simulink model "FOC_2"  (R2024a)
settings: Solver=FixedStepAuto  StartTime=0.0  StopTime=Inf  RelTol=1e-3  EnableMultiTasking=on
undefined symbols (not defined in the file): DiscIntNeverNeededParam, Down, GPTRIP1SEL, Ki, Ki_s, Kp, Kp_s, L, lambda, ma, p, T_period, TZ1, Up, Vdc
libraries: eeGeneralControl x6, simulink x6, c2837xDlib x5, c2802xlib x3
settings Model: ExtModeTrigDuration=8  Creator=kareem  LastModifiedBy=kareem
settings SolverCC: AutoInsertRateTranBlk=on
settings OptimizationCC: DefaultUnderspecifiedDataType=single  EnhancedBackFolding=on  PassReuseOutputArgsAs=Individual arguments  MaxStackSize=1024  OptimizeBlockOrder=speed  DifferentSizesBufferReuse=on  OptimizationCustomize=off  EfficientTunableParamExpr=on
settings DebuggingCC: MultiTaskRateTransMsg=warning  ParameterTunabilityLossMsg=error
settings HardwareCC: ProdBitPerChar=16  ProdBitPerInt=16  ProdBitPerPointer=32  ProdBitPerSizeT=32  ProdBitPerPtrDiffT=32  ProdLargestAtomicInteger=Integer  ProdLargestAtomicFloat=None  ProdWordSize=16  ProdLongLongMode=on  ProdHWDeviceType=Texas Instruments->C2000  HardwareBoardFeatureSet=SoCBlockset
settings SFSimCC: MATLABDynamicMemAlloc=off
settings RTWCC: Description=Embedded Coder  SystemTargetFile=ert.tlc  HardwareBoard=TI Delfino F28379D LaunchPad  TemplateMakefile=ert_default_tmf  Toolchain=Texas Instruments Code Composer Studio (C2000)  CodeProfilingSaveOptions=MetricsOnly
settings CodeAppCC: ForceParamTrailComments=on  IgnoreCustomStorageClasses=off  OperatorAnnotations=on  SimulinkDataObjDesc=on  SFDataObjDesc=on  InsertBlockDesc=on
settings ERTTargetCC: CodeReplacementLibrary=TI C28x  ExtModeTransport=4  ExtModeStaticAlloc=on  ExtModeAutomaticAllocSize=off  ExtModeStaticAllocSize=10000  ExtModeMexFile=ext_xcp  ExtModeIntrfLevel=Level2 - Open

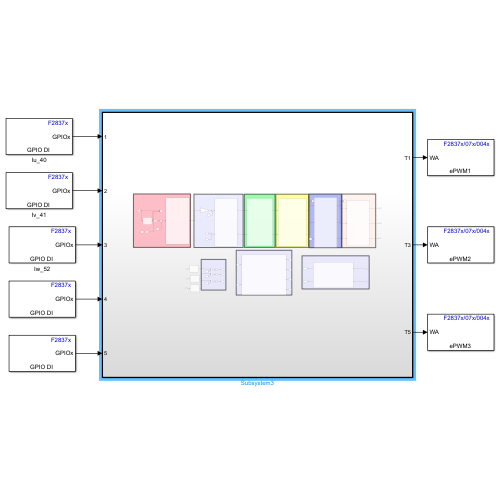
[thumbnail: Simulink's stored preview of the top-level diagram]
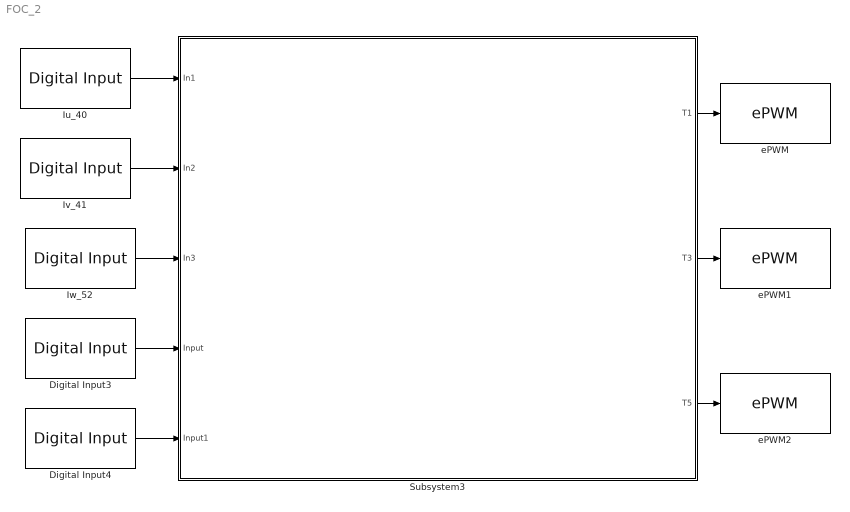
== system FOC_2 ==
  Digital Input3 : c2837xDlib/Digital Input  GPIO_Number=GPIO64~GPIO71  GPIO_Bit0=off  GPIO_Bit1=on  GPIO_Bit2=off  GPIO_Bit3=off  GPIO_Bit4=off  GPIO_Bit5=off  GPIO_Bit6=off  GPIO_Bit7=off  sampleTime=0.1  dataType=auto  GPIO_Bit0_Qualification=Sync to SYSCLKOUT  GPIO_Bit1_Qualification=Sync to SYSCLKOUT  GPIO_Bit2_Qualification=Sync to SYSCLKOUT  GPIO_Bit3_Qualification=Sync to SYSCLKOUT  GPIO_Bit4_Qualification=Sync to SYSCLKOUT  GPIO_Bit5_Qualification=Sync to SYSCLKOUT  GPIO_Bit6_Qualification=Sync to SYSCLKOUT  GPIO_Bit7_Qualification=Sync to SYSCLKOUT  Qualification_Period=-1
  Digital Input4 : c2837xDlib/Digital Input  GPIO_Number=GPIO88~GPIO95  GPIO_Bit0=off  GPIO_Bit1=off  GPIO_Bit2=off  GPIO_Bit3=off  GPIO_Bit4=off  GPIO_Bit5=off  GPIO_Bit6=on  GPIO_Bit7=off  sampleTime=0.1  dataType=auto  GPIO_Bit0_Qualification=Sync to SYSCLKOUT  GPIO_Bit1_Qualification=Sync to SYSCLKOUT  GPIO_Bit2_Qualification=Sync to SYSCLKOUT  GPIO_Bit3_Qualification=Sync to SYSCLKOUT  GPIO_Bit4_Qualification=Sync to SYSCLKOUT  GPIO_Bit5_Qualification=Sync to SYSCLKOUT  GPIO_Bit6_Qualification=Sync to SYSCLKOUT  GPIO_Bit7_Qualification=Sync to SYSCLKOUT  Qualification_Period=-1
  Iu_40 : c2837xDlib/Digital Input  GPIO_Number=GPIO40~GPIO47  GPIO_Bit0=on  GPIO_Bit1=off  GPIO_Bit2=off  GPIO_Bit3=off  GPIO_Bit4=off  GPIO_Bit5=off  GPIO_Bit6=off  GPIO_Bit7=off  sampleTime=0.1  dataType=auto  GPIO_Bit0_Qualification=Sync to SYSCLKOUT  GPIO_Bit1_Qualification=Sync to SYSCLKOUT  GPIO_Bit2_Qualification=Sync to SYSCLKOUT  GPIO_Bit3_Qualification=Sync to SYSCLKOUT  GPIO_Bit4_Qualification=Sync to SYSCLKOUT  GPIO_Bit5_Qualification=Sync to SYSCLKOUT  GPIO_Bit6_Qualification=Sync to SYSCLKOUT  GPIO_Bit7_Qualification=Sync to SYSCLKOUT  Qualification_Period=-1
  Iv_41 : c2837xDlib/Digital Input  GPIO_Number=GPIO40~GPIO47  GPIO_Bit0=off  GPIO_Bit1=on  GPIO_Bit2=off  GPIO_Bit3=off  GPIO_Bit4=off  GPIO_Bit5=off  GPIO_Bit6=off  GPIO_Bit7=off  sampleTime=0.1  dataType=auto  GPIO_Bit0_Qualification=Sync to SYSCLKOUT  GPIO_Bit1_Qualification=Sync to SYSCLKOUT  GPIO_Bit2_Qualification=Sync to SYSCLKOUT  GPIO_Bit3_Qualification=Sync to SYSCLKOUT  GPIO_Bit4_Qualification=Sync to SYSCLKOUT  GPIO_Bit5_Qualification=Sync to SYSCLKOUT  GPIO_Bit6_Qualification=Sync to SYSCLKOUT  GPIO_Bit7_Qualification=Sync to SYSCLKOUT  Qualification_Period=-1
  Iw_52 : c2837xDlib/Digital Input  GPIO_Number=GPIO48~GPIO55  GPIO_Bit0=off  GPIO_Bit1=off  GPIO_Bit2=off  GPIO_Bit3=off  GPIO_Bit4=on  GPIO_Bit5=off  GPIO_Bit6=off  GPIO_Bit7=off  sampleTime=0.1  dataType=auto  GPIO_Bit0_Qualification=Sync to SYSCLKOUT  GPIO_Bit1_Qualification=Sync to SYSCLKOUT  GPIO_Bit2_Qualification=Sync to SYSCLKOUT  GPIO_Bit3_Qualification=Sync to SYSCLKOUT  GPIO_Bit4_Qualification=Sync to SYSCLKOUT  GPIO_Bit5_Qualification=Sync to SYSCLKOUT  GPIO_Bit6_Qualification=Sync to SYSCLKOUT  GPIO_Bit7_Qualification=Sync to SYSCLKOUT  Qualification_Period=-1
  Subsystem3 : Subsystem  TreatAsAtomicUnit=on
  ePWM : c2802xlib/ePWM  PwmType=C2000_Type4  useModule=ePWM1  ePWMxLINKTBPRD=Not Linked  periodUnits=Clock cycles  timerSource=Specify via dialog  timerPeriod_clk=10000  timerPeriod_sec=0.0001  tbshadow=Counter equals to zero  countingMode=Up-Down  phaseActiveEnable=Disable  phaseDirection=Count down after sync  phaseActive=0  synchronizationEnable=off  dcaevt1Sync=off  dcbevt1Sync=off  synchronizationOption=Disable  dcbevt1SyncOut=off  dcaevt1SyncOut=off  cmpdSyncOut=off  cmpcSyncOut=off  cmpbSyncOut=off  zeroSyncOut=off  swfSyncOut=off  perSynchronizationOption=Counter equals to period (CTR=PRD)  clockPrescale=1  HSclockPrescale=1  enswap=off  ePWMxAStatus=on  ePWMxAactionLogic1=Do nothing  ePWMxAactionLogic2=Do nothing  ePWMxAactionLogic3=Clear  ePWMxAactionLogic4=Set  ePWMxAactionLogic5=Do nothing  ePWMxAactionLogic6=Do nothing  ePWMxACSFenable=off  ePWMxACSFvalue=Forcing disable  ePWMxASFreload=Zero  ePWMxBStatus=on  ePWMxBactionLogic1=Do nothing  ePWMxBactionLogic2=Do nothing  ePWMxBactionLogic3=Set  ePWMxBactionLogic4=Clear  ePWMxBactionLogic5=Do nothing  ePWMxBactionLogic6=Do nothing  ePWMxBCSFenable=off  ePWMxBCSFvalue=Forcing disable  ePWMxBSFreload=Zero  ePWNxBOutWay=off  ePWMxLINKCMPA=Not Linked  CMPAUnits=Clock cycles  CMPASource=Input port  CMPAValue_per=50  CMPAValue_clk=0  enCMPAshadow=Counter equals to zero (CTR=Zero)  ePWMxLINKCMPB=Not Linked  CMPBUnits=Clock cycles  CMPBSource=Specify via dialog  CMPBValue_per=50  CMPBValue_clk=32000  enCMPBshadow=Counter equals to zero (CTR=Zero)  ePWMxLINKCMPC=Not Linked  CMPCUnits=Clock cycles  CMPCSource=Specify via dialog  CMPCValue_per=50  CMPCValue_clk=32000  enCMPCshadow=Counter equals to zero (CTR=Zero)  ePWMxLINKCMPD=Not Linked  CMPDUnits=Clock cycles  CMPDSource=Specify via dialog  CMPDValue_per=50  CMPDValue_clk=32000  enCMPDshadow=Counter equals to zero (CTR=Zero)  enableDBePWMxA=on  enableDBePWMxB=on  enhalfcycle=off  DBpolarity=Active high complementary (AHC)  DBedgeDelay=Positive  DBSource_ePWMxA=ePWMxA  DBSource_ePWMxB=ePWMxA  DBPeriodUnits=Clock cycles  DBperiodSource=Specify via dialog  REDperiod=400  FEDperiod=400  REDperiod_sec=0  FEDperiod_sec=0  LoadModeDBRED=Immediate without using shadow  LoadModeDBFED=Immediate without using shadow  adcstartModuleA=off  adcrequestEventA=First event  adcstartEventA=Digital Compare Module A Event 1 start of conversion (DCAEVT1.soc)  adcstartEventA_type2=Counter equals to zero (CTR=Zero)  adcstartModuleB=off  adcrequestEventB=First event  adcstartEventB=Counter equals to zero (CTR=Zero)  adcstartEventB_type2=Counter equals to zero (CTR=Zero)  intEn=off  intPrd=First event  intSel=Counter equals to zero (CTR=Zero)  intSel_type2=Counter equals to zero (CTR=Zero)  hrpe=off  enHRPWM=off  HRPWM_LoadMode=Counter equals to period (CTR=PRD)  HRPWM_CTLMode=Duty or Period control mode  HRPWM_EDGMode=Both edge  hrpeb=off  enHRPWMB=off  HRPWM_LoadModeB=Counter equals to zero (CTR=ZERO)  HRPWM_CTLModeB=Duty or Period control mode  HRPWM_EDGModeB=Both edge  enHRDBRED=off  enHRDBFED=off  enSFO=on  enautoconv=on  chopperEnable=off  chopperFrequency=1  chopperFirstwidth=1  chopperDuty=12.5%  tripZonesource=Specify via dialog  tzselOSHT1=off  tzselOSHT2=off  tzselOSHT3=off  tzselOSHT4=off  tzselOSHT5=off  tzselOSHT6=off  tzselOSHDCAEV1=off  tzselOSHDCBEV1=off  tzselCBC1=off  tzselCBC2=off  tzselCBC3=off  tzselCBC4=off  tzselCBC5=off  tzselCBC6=off  tzselCBCDCAEV2=off  tzselCBCDCBEV2=off  enTzOstIntr=off  enTzCbcIntr=off  enTzDCAEVT1Intr=off  enTzDCAEVT2Intr=off  enTzDCBEVT1Intr=off  enTzDCBEVT2Intr=off  tzclrCBCLatch=Counter equals to zero (CTR=Zero)  ePWMxAforced=No action  ePWMxBforced=No action  DCAEVT1forced=No action  DCBEVT1forced=No action  DCAEVT2forced=No action  DCBEVT2forced=No action  dcah=Trip Zone 1 input (TZ1)  dcal=Trip Zone 2 input (TZ2)  dcbh=Trip Zone 1 input (TZ1)  dcbl=Trip Zone 2 input (TZ2)  dcah_type2=GPTRIP1SEL/(TZ1)  dcal_type2=GPTRIP1SEL/(TZ1)  dcbh_type2=GPTRIP1SEL/(TZ1)  dcbl_type2=GPTRIP1SEL/(TZ1)  gendcaevt1=Event disabled  gendcaevt2=Event disabled  gendcbevt1=Event disabled  gendcbevt2=Event disabled  dcaevt1src=DCAEVT1 with sync  dcaevt2src=DCAEVT2 with sync  dcbevt1src=DCBEVT1 with sync  dcbevt2src=DCBEVT2 with sync  pulsesel=Counter equals to zero (CTR=Zero)  blankinv=off  blankoffset=0  blankwidth=0  evsrcsel=Filtered version of DCAEVT1 (DCAEVT1FILT)  encape=off
      settings: LibrarySourceBlock=c2837xDlib/ePWM
  ePWM1 : c2802xlib/ePWM  PwmType=C2000_Type4  useModule=ePWM2  ePWMxLINKTBPRD=Not Linked  periodUnits=Clock cycles  timerSource=Specify via dialog  timerPeriod_clk=10000  timerPeriod_sec=0.0001  tbshadow=Counter equals to zero  countingMode=Up-Down  phaseActiveEnable=Disable  phaseDirection=Count down after sync  phaseActive=0  synchronizationEnable=off  dcaevt1Sync=off  dcbevt1Sync=off  synchronizationOption=Disable  dcbevt1SyncOut=off  dcaevt1SyncOut=off  cmpdSyncOut=off  cmpcSyncOut=off  cmpbSyncOut=off  zeroSyncOut=off  swfSyncOut=off  perSynchronizationOption=Counter equals to period (CTR=PRD)  clockPrescale=1  HSclockPrescale=1  enswap=off  ePWMxAStatus=on  ePWMxAactionLogic1=Do nothing  ePWMxAactionLogic2=Do nothing  ePWMxAactionLogic3=Clear  ePWMxAactionLogic4=Set  ePWMxAactionLogic5=Do nothing  ePWMxAactionLogic6=Do nothing  ePWMxACSFenable=off  ePWMxACSFvalue=Forcing disable  ePWMxASFreload=Zero  ePWMxBStatus=on  ePWMxBactionLogic1=Do nothing  ePWMxBactionLogic2=Do nothing  ePWMxBactionLogic3=Set  ePWMxBactionLogic4=Clear  ePWMxBactionLogic5=Do nothing  ePWMxBactionLogic6=Do nothing  ePWMxBCSFenable=off  ePWMxBCSFvalue=Forcing disable  ePWMxBSFreload=Zero  ePWNxBOutWay=off  ePWMxLINKCMPA=Not Linked  CMPAUnits=Clock cycles  CMPASource=Input port  CMPAValue_per=50  CMPAValue_clk=0  enCMPAshadow=Counter equals to zero (CTR=Zero)  ePWMxLINKCMPB=Not Linked  CMPBUnits=Clock cycles  CMPBSource=Specify via dialog  CMPBValue_per=50  CMPBValue_clk=32000  enCMPBshadow=Counter equals to zero (CTR=Zero)  ePWMxLINKCMPC=Not Linked  CMPCUnits=Clock cycles  CMPCSource=Specify via dialog  CMPCValue_per=50  CMPCValue_clk=32000  enCMPCshadow=Counter equals to zero (CTR=Zero)  ePWMxLINKCMPD=Not Linked  CMPDUnits=Clock cycles  CMPDSource=Specify via dialog  CMPDValue_per=50  CMPDValue_clk=32000  enCMPDshadow=Counter equals to zero (CTR=Zero)  enableDBePWMxA=on  enableDBePWMxB=on  enhalfcycle=off  DBpolarity=Active high complementary (AHC)  DBedgeDelay=Positive  DBSource_ePWMxA=ePWMxA  DBSource_ePWMxB=ePWMxA  DBPeriodUnits=Clock cycles  DBperiodSource=Specify via dialog  REDperiod=400  FEDperiod=400  REDperiod_sec=0  FEDperiod_sec=0  LoadModeDBRED=Immediate without using shadow  LoadModeDBFED=Immediate without using shadow  adcstartModuleA=off  adcrequestEventA=First event  adcstartEventA=Digital Compare Module A Event 1 start of conversion (DCAEVT1.soc)  adcstartEventA_type2=Counter equals to zero (CTR=Zero)  adcstartModuleB=off  adcrequestEventB=First event  adcstartEventB=Counter equals to zero (CTR=Zero)  adcstartEventB_type2=Counter equals to zero (CTR=Zero)  intEn=off  intPrd=First event  intSel=Counter equals to zero (CTR=Zero)  intSel_type2=Counter equals to zero (CTR=Zero)  hrpe=off  enHRPWM=off  HRPWM_LoadMode=Counter equals to period (CTR=PRD)  HRPWM_CTLMode=Duty or Period control mode  HRPWM_EDGMode=Both edge  hrpeb=off  enHRPWMB=off  HRPWM_LoadModeB=Counter equals to zero (CTR=ZERO)  HRPWM_CTLModeB=Duty or Period control mode  HRPWM_EDGModeB=Both edge  enHRDBRED=off  enHRDBFED=off  enSFO=on  enautoconv=on  chopperEnable=off  chopperFrequency=1  chopperFirstwidth=1  chopperDuty=12.5%  tripZonesource=Specify via dialog  tzselOSHT1=off  tzselOSHT2=off  tzselOSHT3=off  tzselOSHT4=off  tzselOSHT5=off  tzselOSHT6=off  tzselOSHDCAEV1=off  tzselOSHDCBEV1=off  tzselCBC1=off  tzselCBC2=off  tzselCBC3=off  tzselCBC4=off  tzselCBC5=off  tzselCBC6=off  tzselCBCDCAEV2=off  tzselCBCDCBEV2=off  enTzOstIntr=off  enTzCbcIntr=off  enTzDCAEVT1Intr=off  enTzDCAEVT2Intr=off  enTzDCBEVT1Intr=off  enTzDCBEVT2Intr=off  tzclrCBCLatch=Counter equals to zero (CTR=Zero)  ePWMxAforced=No action  ePWMxBforced=No action  DCAEVT1forced=No action  DCBEVT1forced=No action  DCAEVT2forced=No action  DCBEVT2forced=No action  dcah=Trip Zone 1 input (TZ1)  dcal=Trip Zone 2 input (TZ2)  dcbh=Trip Zone 1 input (TZ1)  dcbl=Trip Zone 2 input (TZ2)  dcah_type2=GPTRIP1SEL/(TZ1)  dcal_type2=GPTRIP1SEL/(TZ1)  dcbh_type2=GPTRIP1SEL/(TZ1)  dcbl_type2=GPTRIP1SEL/(TZ1)  gendcaevt1=Event disabled  gendcaevt2=Event disabled  gendcbevt1=Event disabled  gendcbevt2=Event disabled  dcaevt1src=DCAEVT1 with sync  dcaevt2src=DCAEVT2 with sync  dcbevt1src=DCBEVT1 with sync  dcbevt2src=DCBEVT2 with sync  pulsesel=Counter equals to zero (CTR=Zero)  blankinv=off  blankoffset=0  blankwidth=0  evsrcsel=Filtered version of DCAEVT1 (DCAEVT1FILT)  encape=off
      settings: LibrarySourceBlock=c2837xDlib/ePWM
  ePWM2 : c2802xlib/ePWM  PwmType=C2000_Type4  useModule=ePWM3  ePWMxLINKTBPRD=Not Linked  periodUnits=Clock cycles  timerSource=Specify via dialog  timerPeriod_clk=10000  timerPeriod_sec=0.0001  tbshadow=Counter equals to zero  countingMode=Up-Down  phaseActiveEnable=Disable  phaseDirection=Count down after sync  phaseActive=0  synchronizationEnable=off  dcaevt1Sync=off  dcbevt1Sync=off  synchronizationOption=Disable  dcbevt1SyncOut=off  dcaevt1SyncOut=off  cmpdSyncOut=off  cmpcSyncOut=off  cmpbSyncOut=off  zeroSyncOut=off  swfSyncOut=off  perSynchronizationOption=Counter equals to period (CTR=PRD)  clockPrescale=1  HSclockPrescale=1  enswap=off  ePWMxAStatus=on  ePWMxAactionLogic1=Do nothing  ePWMxAactionLogic2=Do nothing  ePWMxAactionLogic3=Clear  ePWMxAactionLogic4=Set  ePWMxAactionLogic5=Do nothing  ePWMxAactionLogic6=Do nothing  ePWMxACSFenable=off  ePWMxACSFvalue=Forcing disable  ePWMxASFreload=Zero  ePWMxBStatus=on  ePWMxBactionLogic1=Do nothing  ePWMxBactionLogic2=Do nothing  ePWMxBactionLogic3=Set  ePWMxBactionLogic4=Clear  ePWMxBactionLogic5=Do nothing  ePWMxBactionLogic6=Do nothing  ePWMxBCSFenable=off  ePWMxBCSFvalue=Forcing disable  ePWMxBSFreload=Zero  ePWNxBOutWay=off  ePWMxLINKCMPA=Not Linked  CMPAUnits=Clock cycles  CMPASource=Input port  CMPAValue_per=50  CMPAValue_clk=0  enCMPAshadow=Counter equals to zero (CTR=Zero)  ePWMxLINKCMPB=Not Linked  CMPBUnits=Clock cycles  CMPBSource=Specify via dialog  CMPBValue_per=50  CMPBValue_clk=32000  enCMPBshadow=Counter equals to zero (CTR=Zero)  ePWMxLINKCMPC=Not Linked  CMPCUnits=Clock cycles  CMPCSource=Specify via dialog  CMPCValue_per=50  CMPCValue_clk=32000  enCMPCshadow=Counter equals to zero (CTR=Zero)  ePWMxLINKCMPD=Not Linked  CMPDUnits=Clock cycles  CMPDSource=Specify via dialog  CMPDValue_per=50  CMPDValue_clk=32000  enCMPDshadow=Counter equals to zero (CTR=Zero)  enableDBePWMxA=on  enableDBePWMxB=on  enhalfcycle=off  DBpolarity=Active high complementary (AHC)  DBedgeDelay=Positive  DBSource_ePWMxA=ePWMxA  DBSource_ePWMxB=ePWMxA  DBPeriodUnits=Clock cycles  DBperiodSource=Specify via dialog  REDperiod=400  FEDperiod=400  REDperiod_sec=0  FEDperiod_sec=0  LoadModeDBRED=Immediate without using shadow  LoadModeDBFED=Immediate without using shadow  adcstartModuleA=off  adcrequestEventA=First event  adcstartEventA=Digital Compare Module A Event 1 start of conversion (DCAEVT1.soc)  adcstartEventA_type2=Counter equals to zero (CTR=Zero)  adcstartModuleB=off  adcrequestEventB=First event  adcstartEventB=Counter equals to zero (CTR=Zero)  adcstartEventB_type2=Counter equals to zero (CTR=Zero)  intEn=off  intPrd=First event  intSel=Counter equals to zero (CTR=Zero)  intSel_type2=Counter equals to zero (CTR=Zero)  hrpe=off  enHRPWM=off  HRPWM_LoadMode=Counter equals to period (CTR=PRD)  HRPWM_CTLMode=Duty or Period control mode  HRPWM_EDGMode=Both edge  hrpeb=off  enHRPWMB=off  HRPWM_LoadModeB=Counter equals to zero (CTR=ZERO)  HRPWM_CTLModeB=Duty or Period control mode  HRPWM_EDGModeB=Both edge  enHRDBRED=off  enHRDBFED=off  enSFO=on  enautoconv=on  chopperEnable=off  chopperFrequency=1  chopperFirstwidth=1  chopperDuty=12.5%  tripZonesource=Specify via dialog  tzselOSHT1=off  tzselOSHT2=off  tzselOSHT3=off  tzselOSHT4=off  tzselOSHT5=off  tzselOSHT6=off  tzselOSHDCAEV1=off  tzselOSHDCBEV1=off  tzselCBC1=off  tzselCBC2=off  tzselCBC3=off  tzselCBC4=off  tzselCBC5=off  tzselCBC6=off  tzselCBCDCAEV2=off  tzselCBCDCBEV2=off  enTzOstIntr=off  enTzCbcIntr=off  enTzDCAEVT1Intr=off  enTzDCAEVT2Intr=off  enTzDCBEVT1Intr=off  enTzDCBEVT2Intr=off  tzclrCBCLatch=Counter equals to zero (CTR=Zero)  ePWMxAforced=No action  ePWMxBforced=No action  DCAEVT1forced=No action  DCBEVT1forced=No action  DCAEVT2forced=No action  DCBEVT2forced=No action  dcah=Trip Zone 1 input (TZ1)  dcal=Trip Zone 2 input (TZ2)  dcbh=Trip Zone 1 input (TZ1)  dcbl=Trip Zone 2 input (TZ2)  dcah_type2=GPTRIP1SEL/(TZ1)  dcal_type2=GPTRIP1SEL/(TZ1)  dcbh_type2=GPTRIP1SEL/(TZ1)  dcbl_type2=GPTRIP1SEL/(TZ1)  gendcaevt1=Event disabled  gendcaevt2=Event disabled  gendcbevt1=Event disabled  gendcbevt2=Event disabled  dcaevt1src=DCAEVT1 with sync  dcaevt2src=DCAEVT2 with sync  dcbevt1src=DCBEVT1 with sync  dcbevt2src=DCBEVT2 with sync  pulsesel=Counter equals to zero (CTR=Zero)  blankinv=off  blankoffset=0  blankwidth=0  evsrcsel=Filtered version of DCAEVT1 (DCAEVT1FILT)  encape=off
      settings: LibrarySourceBlock=c2837xDlib/ePWM
  wires:
  Subsystem3/1(T1) -> ePWM/1
  Subsystem3/2(T3) -> ePWM1/1
  Subsystem3/3(T5) -> ePWM2/1
  Iw_52/1 -> Subsystem3/3(In3)
  Iv_41/1 -> Subsystem3/2(In2)
  Iu_40/1 -> Subsystem3/1(In1)
  Digital Input3/1 -> Subsystem3/4(Input)
  Digital Input4/1 -> Subsystem3/5(Input1)

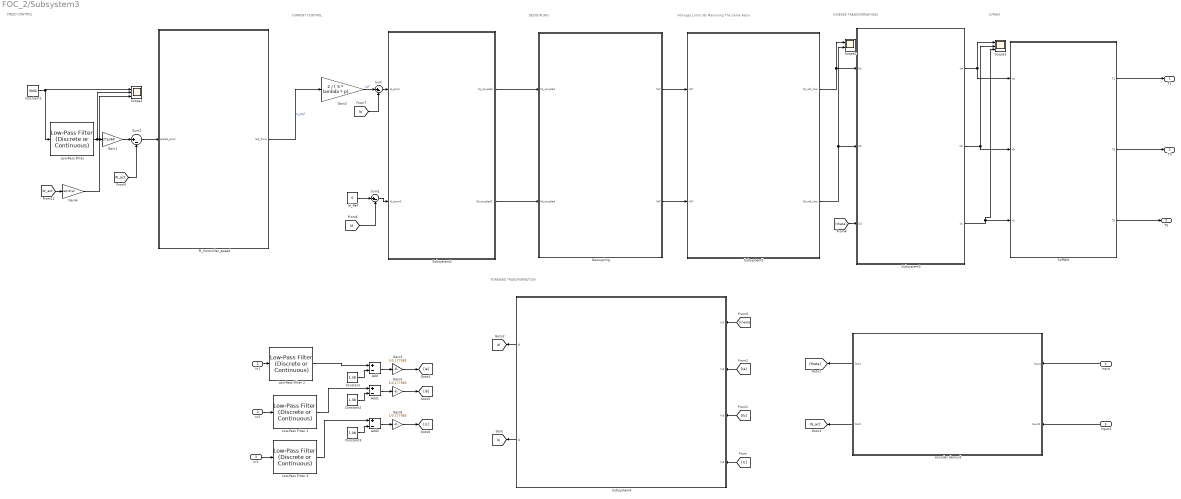
== system FOC_2/Subsystem3 ==
  note: Voltages Limits By Maintaing The Same Ratio
  note: FORWARD TRANSFORMATION
  note: SPEED CONTROL
  note: CURRENT CONTROL
  note: DECOUPLING
  note: INVERSE TRANSFORMATIONS
  note: SVPWM
  In1 : Inport
  In2 : Inport  Port=2
  In3 : Inport  Port=3
  Input : Inport  Port=4
  Input1 : Inport  Port=5
  Add : Sum  Inputs=+-
  Add1 : Sum  Inputs=+-
  Add2 : Sum  Inputs=+-
  Constant : Constant  Value=1.38
  Constant1 : Constant  Value=3000
  Constant2 : Constant  Value=1.38
  Constant3 : Constant  Value=1.38
  Decoupling : Subsystem
  Gain1 : Gain  Gain=2*pi/60
  Gain2 : Gain  Gain=2 / ( 3 * lambda * p)
  Gain3 : Gain  Gain=1/0.177985
  Gain4 : Gain  Gain=60/(2*pi)
  Gain5 : Gain  Gain=1/0.177985
  Gain6 : Gain  Gain=1/0.177985
  Id_Ref : Constant  Value=0
  Low-Pass Filter {,1..3} (4 alike) : eeGeneralControl/Low-Pass Filter (Discrete or Continuous)  K=1  T=1/100  B=inf  A=-inf  init_option=Inherited from block input  x0=0  Ts=-1
  PI_Controller_speed : Subsystem
  SVPWM : Subsystem
  Scope1 : Scope  NumInputPorts=3
  Scope3 : Scope  NumInputPorts=3
  Scope4 : Scope  NumInputPorts=2
  Subsystem2 : Subsystem
  Subsystem3 : Subsystem
  Subsystem4 : Subsystem
  Subsystem5 : Subsystem
  Sum : Sum  Inputs=|+-
  Sum1 : Sum  Inputs=|+-
  Sum2 : Sum  Inputs=|+-
  encoder demux1 : Subsystem
  T1 : Outport
  T3 : Outport  Port=2
  T5 : Outport  Port=3
  tag scope: Id=global, Iq=global, W_act=global
  wires:
  Gain4/1 -> Scope1/3
  Sum/1 -> Subsystem2/1(Iq_error)
  Constant1/1 -> "Low-Pass Filter "/1, Scope1/1
  Subsystem2/2(Vd_coupled1) -> Decoupling/2(Vd_coupled)
  Gain1/1 -> Sum2/1
  [Id] -> Sum1/2
  Decoupling/1(Vq*) -> Subsystem5/1(Vq*)
  Decoupling/2(Vd*) -> Subsystem5/2(Vd*)
  "Low-Pass Filter "/1 -> Scope1/2, Gain1/1
  Subsystem3/2(Vb) -> SVPWM/2(Vb), Scope3/2
  Subsystem4/2(Iq) -> [Iq]
  Sum1/1 -> Subsystem2/2(Id_error1)
  Subsystem2/1(Vq_coupled) -> Decoupling/1(Vq_coupled)
  PI_Controller_speed/1(req_Torq) -> Gain2/1  "Iq_Ref"
  Subsystem5/2(Vd_ref_new) -> Subsystem3/2(Vd), Scope4/2
  Gain2/1 -> Sum/1  "I_q*"
  [W_act] -> Gain4/1
  Subsystem4/1(Id) -> [Id]
  Subsystem3/3(Vc) -> Scope3/3, SVPWM/3(Vc)
  Subsystem3/1(Va) -> Scope3/1, SVPWM/1(Va)
  Subsystem5/1(Vq_ref_new) -> Scope4/1, Subsystem3/1(Vq)
  Id_Ref/1 -> Sum1/1
  [Ic] -> Subsystem4/4(In4)
  [W_act] -> Sum2/2
  SVPWM/1(T1) -> T1/1
  [Iq] -> Sum/2
  Sum2/1 -> PI_Controller_speed/1(speed_error)
  [Ib] -> Subsystem4/3(In3)
  [theta] -> Subsystem4/1(In1)
  [Ia] -> Subsystem4/2(In2)
  [theta] -> Subsystem3/3(In2)
  SVPWM/3(T5) -> T5/1
  SVPWM/2(T3) -> T3/1
  Input/1 -> encoder demux1/1(Input)
  Input1/1 -> encoder demux1/2(Input1)
  encoder demux1/1(Out1) -> [theta]
  encoder demux1/2(Out2) -> [W_act]
  Add/1 -> Gain3/1
  Constant/1 -> Add/2
  Gain3/1 -> [Ia]
  Constant2/1 -> Add1/2
  Add1/1 -> Gain5/1
  Add2/1 -> Gain6/1
  Constant3/1 -> Add2/2
  Gain5/1 -> [Ib]
  Gain6/1 -> [Ic]
  In1/1 -> Low-Pass Filter 2/1
  In2/1 -> Low-Pass Filter 1/1
  In3/1 -> Low-Pass Filter 3/1
  Low-Pass Filter 2/1 -> Add/1
  Low-Pass Filter 1/1 -> Add1/1
  Low-Pass Filter 3/1 -> Add2/1

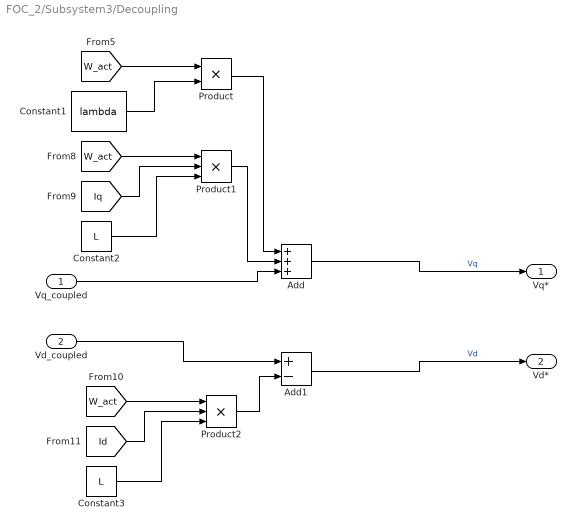
== system FOC_2/Subsystem3/Decoupling ==
  Vq_coupled : Inport
  Vd_coupled : Inport  Port=2
  Add : Sum  Inputs=+++
  Add1 : Sum  Inputs=+-
  Constant1 : Constant  Value=lambda
  Constant2 : Constant  Value=L
  Constant3 : Constant  Value=L
  Product : Product
  Product1 : Product  Inputs=3
  Product2 : Product  Inputs=3
  Vq* : Outport
  Vd* : Outport  Port=2
  wires:
  [W_act] -> Product1/1
  Product/1 -> Add/1
  Product1/1 -> Add/2
  [W_act] -> Product2/1
  Product2/1 -> Add1/2
  Constant3/1 -> Product2/3
  Constant2/1 -> Product1/3
  Constant1/1 -> Product/2
  [Id] -> Product2/2
  [W_act] -> Product/1
  [Iq] -> Product1/2
  Vd_coupled/1 -> Add1/1
  Add1/1 -> Vd*/1  "Vd"
  Add/1 -> Vq*/1  "Vq"
  Vq_coupled/1 -> Add/3

== system FOC_2/Subsystem3/PI_Controller_speed ==
  speed_error : Inport
  Abs : Abs  SaturateOnIntegerOverflow=off
  Add : Sum
  Add1 : Sum  Inputs=+-
  Compare To Constant1 : simulink/Logic and Bit Operations/Compare To Constant  relop=<=  const=1e-4  OutDataTypeStr=boolean
  Gain3 : Gain  Gain=Kp_s
  Gain4 : Gain  Gain=Ki_s
  Integrator (Discrete or Continuous) : eeGeneralControl/Integrator (Discrete or Continuous)  LabelModeActiveChoice=Discrete  ExternalReset=level  LimitType=Anti-windup  B=4  A=-inf  Ts=-1
  Product : Product
  Saturation : Saturate  UpperLimit=3.8  LowerLimit=-3.8
  req_Torq : Outport
  wires:
  Saturation/1 -> Add1/2, req_Torq/1
  Add/1 -> Add1/1, Saturation/1
  Gain3/1 -> Add/1
  Integrator (Discrete or Continuous)/1 -> Add/2
  Gain4/1 -> Product/1
  Add1/1 -> Abs/1
  Abs/1 -> Compare To Constant1/1
  speed_error/1 -> Gain3/1, Gain4/1
  Product/1 -> Integrator (Discrete or Continuous)/1
  Compare To Constant1/1 -> Product/2

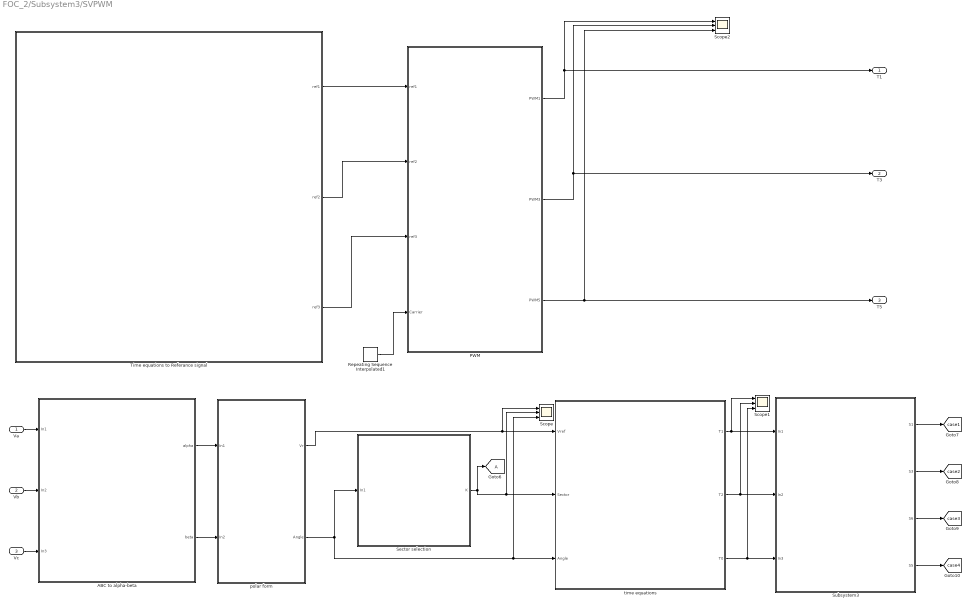
== system FOC_2/Subsystem3/SVPWM ==
  Va : Inport
  Vb : Inport  Port=2
  Vc : Inport  Port=3
  ABC to alpha-beta : Subsystem
  Goto6 : Goto  TagVisibility=global
  PWM : Subsystem
  Repeating Sequence Interpolated1 : simulink/Sources/Repeating Sequence Interpolated  OutValues="[ 0 1/15000  1e-6  ]"  TimeValues=[ 0 1/40000 1/20001]  LookUpMeth=Interpolation-Use End Values  tsamp=1e-6  OutMin=[]  OutMax=[]  OutDataTypeStr=double  OutputDataTypeScalingMode=double  OutDataType=fixdt(0,8)  OutScaling=2^-10
  Scope : Scope  NumInputPorts=3
  Scope1 : Scope  NumInputPorts=3
  Scope2 : Scope  NumInputPorts=3
  Sector selection : Subsystem
  Subsystem3 : Subsystem
  Time equations to Referance signal : Subsystem
  polar form : Subsystem
  time equations : Subsystem
  T1 : Outport
  T3 : Outport  Port=2
  T5 : Outport  Port=3
  tag scope: case1=global, case2=global, case3=global, case4=global
  wires:
  Vb/1 -> ABC to alpha-beta/2(In2)
  time equations/1(T1) -> Scope1/1, Subsystem3/1(In1)
  Va/1 -> ABC to alpha-beta/1(In1)
  Time equations to Referance signal/1(ref1) -> PWM/1(ref1)
  Time equations to Referance signal/2("ref2 ") -> PWM/2(ref2)
  Time equations to Referance signal/3(ref3) -> PWM/3(ref3)
  Vc/1 -> ABC to alpha-beta/3(In3)
  ABC to alpha-beta/1(alpha) -> polar form/1(In1)
  ABC to alpha-beta/2(beta) -> polar form/2(In2)
  PWM/1(PWM1) -> T1/1, Scope2/1
  PWM/2(PWM3) -> T3/1, Scope2/2
  PWM/3(PWM5) -> T5/1, Scope2/3
  polar form/2(Angle) -> Sector selection/1(In1), time equations/3(Angle), Scope/3
  polar form/1(Vr) -> Scope/1, time equations/1(Vref)
  Sector selection/1(K) -> Scope/2, time equations/2(Sector), Goto6/1
  Subsystem3/2(S3) -> [case2]
  Subsystem3/1(S1) -> [case1]
  time equations/3(T0) -> Subsystem3/3(In3), Scope1/3
  time equations/2(T2) -> Scope1/2, Subsystem3/2(In2)
  Subsystem3/4(S5) -> [case4]
  Subsystem3/3(S6) -> [case3]
  Repeating Sequence Interpolated1/1 -> PWM/4(Carrier)

== system FOC_2/Subsystem3/Subsystem2 ==
  Iq_error : Inport
  Id_error1 : Inport  Port=2
  PI_Controller_Id : Subsystem
  PI_Controller_Iq : Subsystem
  Vq_coupled : Outport
  Vd_coupled1 : Outport  Port=2
  wires:
  PI_Controller_Id/1(Vd_coupled) -> Vd_coupled1/1
  Id_error1/1 -> PI_Controller_Id/1(Id_error)
  Iq_error/1 -> PI_Controller_Iq/1(Iq_error)
  PI_Controller_Iq/1(Vq_coupled) -> Vq_coupled/1

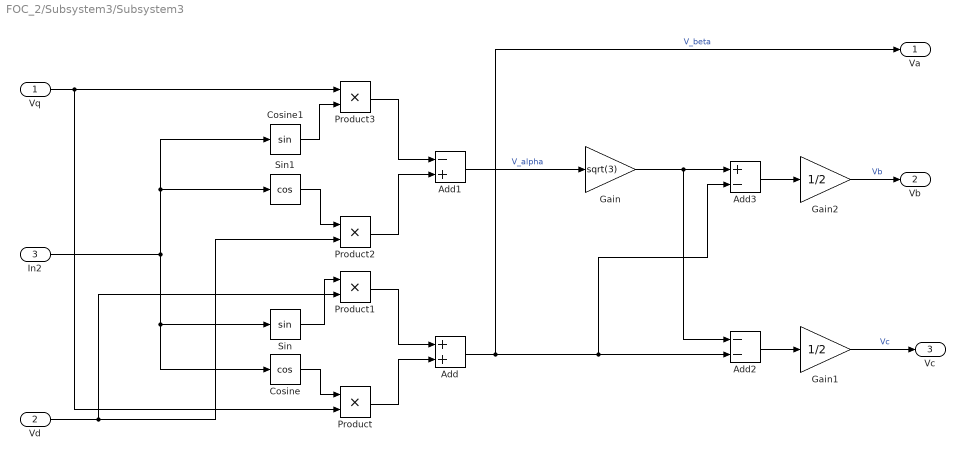
== system FOC_2/Subsystem3/Subsystem3 ==
  Vq : Inport
  Vd : Inport  Port=2
  In2 : Inport  Port=3
  Add : Sum
  Add1 : Sum  Inputs=-+
  Add2 : Sum  Inputs=--
  Add3 : Sum  Inputs=+-
  Cosine : Trigonometry  Operator=cos
  Cosine1 : Trigonometry
  Gain : Gain  Gain=sqrt(3)
  Gain1 : Gain  Gain=1/2
  Gain2 : Gain  Gain=1/2
  Product{,1..3} (4 alike) : Product
  Sin : Trigonometry
  Sin1 : Trigonometry  Operator=cos
  Va : Outport
  Vb : Outport  Port=2
  Vc : Outport  Port=3
  wires:
  Add/1 -> Add3/2, Add2/2, Va/1  "V_beta"
  Product2/1 -> Add1/2
  Product3/1 -> Add1/1
  Cosine/1 -> Product/1
  Sin1/1 -> Product2/1
  Sin/1 -> Product1/1
  Product/1 -> Add/2
  Vd/1 -> Product1/2, Product2/2
  In2/1 -> Sin/1, Cosine/1, Cosine1/1, Sin1/1
  Product1/1 -> Add/1
  Cosine1/1 -> Product3/2
  Add1/1 -> Gain/1  "V_alpha"
  Vq/1 -> Product3/1, Product/2
  Gain1/1 -> Vc/1  "Vc"
  Add3/1 -> Gain2/1
  Gain/1 -> Add2/1, Add3/1
  Add2/1 -> Gain1/1
  Gain2/1 -> Vb/1  "Vb"

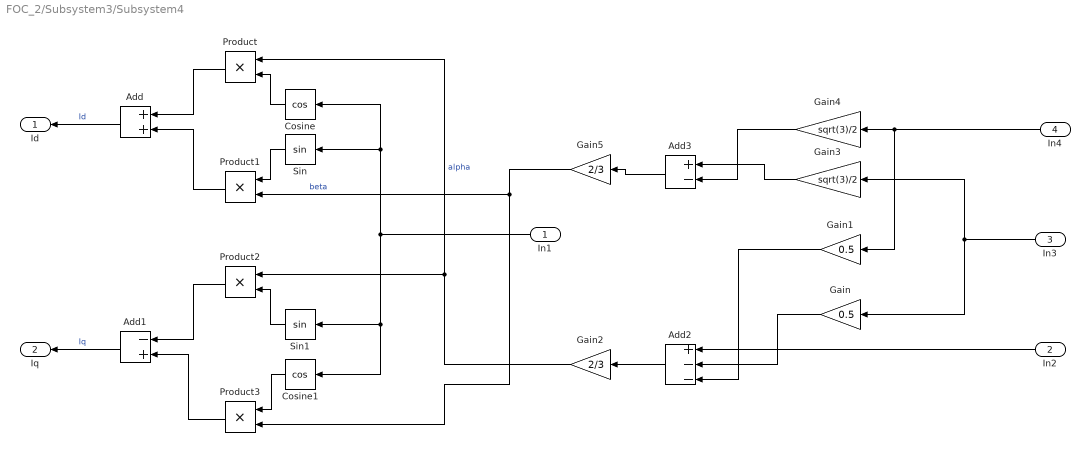
== system FOC_2/Subsystem3/Subsystem4 ==
  In1 : Inport
  In2 : Inport  Port=2
  In3 : Inport  Port=3
  In4 : Inport  Port=4
  Add : Sum
  Add1 : Sum  Inputs=-+
  Add2 : Sum  Inputs=+--
  Add3 : Sum  Inputs=+-
  Cosine : Trigonometry  Operator=cos
  Cosine1 : Trigonometry  Operator=cos
  Gain : Gain  Gain=0.5
  Gain1 : Gain  Gain=0.5
  Gain2 : Gain  Gain=2/3
  Gain3 : Gain  Gain=sqrt(3)/2
  Gain4 : Gain  Gain=sqrt(3)/2
  Gain5 : Gain  Gain=2/3
  Product{,1..3} (4 alike) : Product
  Sin : Trigonometry
  Sin1 : Trigonometry
  Id : Outport
  Iq : Outport  Port=2
  wires:
  Add1/1 -> Iq/1  "Iq"
  Add/1 -> Id/1  "Id"
  Product3/1 -> Add1/2
  Product1/1 -> Add/2
  Sin1/1 -> Product2/2
  Sin/1 -> Product1/1
  Product/1 -> Add/1
  Cosine1/1 -> Product3/1
  In1/1 -> Cosine/1, Sin/1, Cosine1/1, Sin1/1
  Product2/1 -> Add1/1
  Cosine/1 -> Product/2
  Gain5/1 -> Product3/2, Product1/2  "beta"
  Gain2/1 -> Product/1, Product2/1  "alpha"
  Add2/1 -> Gain2/1
  In2/1 -> Add2/1
  Gain/1 -> Add2/2
  In4/1 -> Gain1/1, Gain4/1
  Gain1/1 -> Add2/3
  Add3/1 -> Gain5/1
  Gain4/1 -> Add3/2
  In3/1 -> Gain/1, Gain3/1
  Gain3/1 -> Add3/1

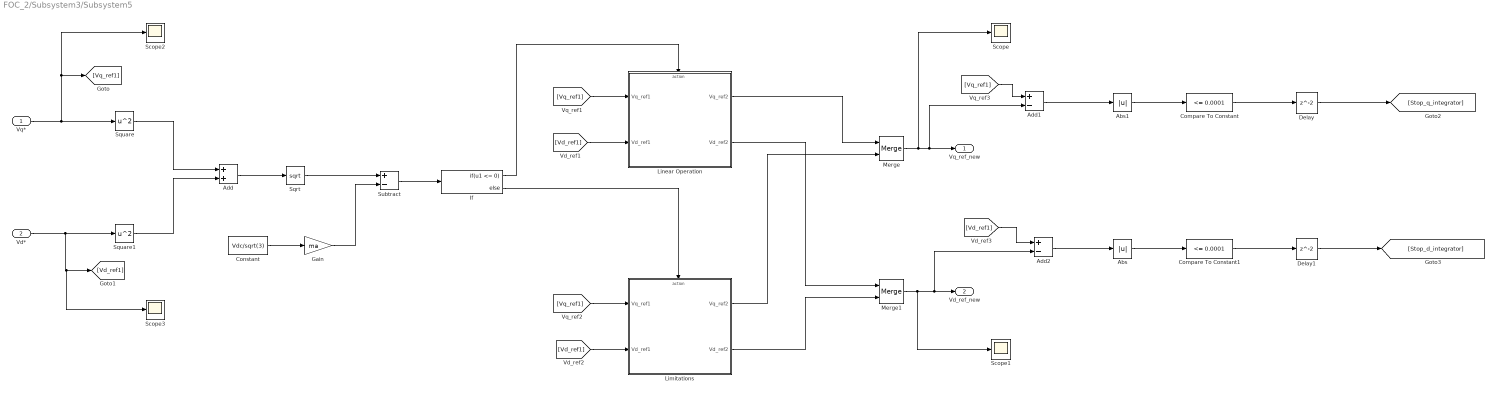
== system FOC_2/Subsystem3/Subsystem5 ==
  Vq* : Inport
  Vd* : Inport  Port=2
  Abs : Abs  SaturateOnIntegerOverflow=off
  Abs1 : Abs  SaturateOnIntegerOverflow=off
  Add : Sum
  Add1 : Sum  Inputs=+-
  Add2 : Sum  Inputs=+-
  Compare To Constant : simulink/Logic and Bit Operations/Compare To Constant  relop=<=  const=0.0001  OutDataTypeStr=boolean
  Compare To Constant1 : simulink/Logic and Bit Operations/Compare To Constant  relop=<=  const=0.0001  OutDataTypeStr=boolean
  Constant : Constant  Value=Vdc/sqrt(3)
  Delay : Delay
  Delay1 : Delay
  Gain : Gain  Gain=ma
  If : If  IfExpression=u1 <= 0
  Limitations : Subsystem  TreatAsAtomicUnit=on
  "Linear Operation " : Subsystem  TreatAsAtomicUnit=on
  Merge : Merge
  Merge1 : Merge
  Scope{,1..3} (4 alike) : Scope
  Sqrt : Sqrt
  Square : Math  Operator=square  SignedPower=on
  Square1 : Math  Operator=square  SignedPower=on
  Subtract : Sum  Inputs=+-
  Vq_ref_new : Outport
  Vd_ref_new : Outport  Port=2
  wires:
  Vd*/1 -> Scope3/1, [Vd_ref1], Square1/1
  Vq*/1 -> Scope2/1, [Vq_ref1], Square/1
  Square/1 -> Add/1
  Square1/1 -> Add/2
  Add/1 -> Sqrt/1
  Constant/1 -> Gain/1
  Sqrt/1 -> Subtract/1
  Gain/1 -> Subtract/2
  Subtract/1 -> If/1
  [Vq_ref1] -> "Linear Operation "/1(Vq_ref1)
  [Vd_ref1] -> "Linear Operation "/2(Vd_ref1)
  If/1 -> "Linear Operation "/Action
  If/2 -> Limitations/Action
  [Vq_ref1] -> Limitations/1(Vq_ref1)
  [Vd_ref1] -> Limitations/2(Vd_ref1)
  Limitations/2(Vd_ref2) -> Merge1/2
  "Linear Operation "/2(Vd_ref2) -> Merge1/1
  Limitations/1(Vq_ref2) -> Merge/2
  "Linear Operation "/1(Vq_ref2) -> Merge/1
  Merge/1 -> Scope/1, Add1/2, Vq_ref_new/1
  Merge1/1 -> Scope1/1, Add2/2, Vd_ref_new/1
  [Vq_ref1] -> Add1/1
  [Vd_ref1] -> Add2/1
  Add2/1 -> Abs/1
  Add1/1 -> Abs1/1
  Abs1/1 -> Compare To Constant/1
  Abs/1 -> Compare To Constant1/1
  Compare To Constant/1 -> Delay/1
  Compare To Constant1/1 -> Delay1/1
  Delay/1 -> [Stop_q_integrator]
  Delay1/1 -> [Stop_d_integrator]

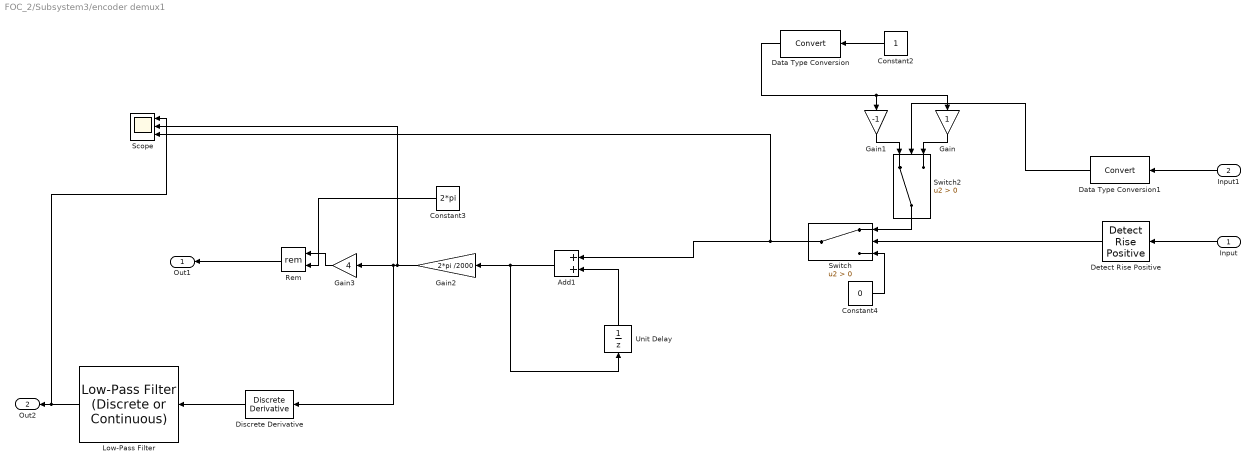
== system FOC_2/Subsystem3/encoder demux1 ==
  Input : Inport
  Input1 : Inport  Port=2
  Add1 : Sum
  Constant2 : Constant
  Constant3 : Constant  Value=2*pi
  Constant4 : Constant  Value=0
  Data Type Conversion : DataTypeConversion  SaturateOnIntegerOverflow=off  RndMeth=Floor
  Data Type Conversion1 : DataTypeConversion  SaturateOnIntegerOverflow=off  RndMeth=Floor
  Detect Rise Positive : simulink/Logic and Bit Operations/Detect Rise Positive  vinit=0  OutDataTypeStr=uint8
  Discrete Derivative : simulink/Discrete/Discrete Derivative  gainval=1.0  ICPrevScaledInput=0.0  OutMin=[]  OutMax=[]  OutDataType=fixdt(1, 16)  OutScaling=2^-10  DoSatur=off
  Gain : Gain
  Gain1 : Gain  Gain=-1
  Gain2 : Gain  Gain=2*pi /2000
  Gain3 : Gain  Gain=4
  "Low-Pass Filter " : eeGeneralControl/Low-Pass Filter (Discrete or Continuous)  K=1  T=1/100  B=inf  A=-inf  init_option=Inherited from block input  x0=0  Ts=-1
  Rem : Math  Operator=rem
  Scope : Scope  NumInputPorts=3
  Switch : Switch  Criteria=u2 > Threshold  SaturateOnIntegerOverflow=off  InputSameDT=off
  Switch2 : Switch  Criteria=u2 > Threshold  SaturateOnIntegerOverflow=off  InputSameDT=off
  Unit Delay : UnitDelay  SampleTime=-1  HasFrameUpgradeWarning=on
  Out1 : Outport
  Out2 : Outport  Port=2
  wires:
  Gain3/1 -> Rem/1
  "Low-Pass Filter "/1 -> Out2/1, Scope/1
  Switch2/1 -> Switch/1
  Gain/1 -> Switch2/3
  Gain1/1 -> Switch2/1
  Data Type Conversion/1 -> Gain1/1, Gain/1
  Constant4/1 -> Switch/3
  Gain2/1 -> Gain3/1, Discrete Derivative/1, Scope/2
  Constant3/1 -> Rem/2
  Data Type Conversion1/1 -> Switch2/2
  Constant2/1 -> Data Type Conversion/1
  Switch/1 -> Add1/1, Scope/3
  Discrete Derivative/1 -> "Low-Pass Filter "/1
  Input/1 -> Detect Rise Positive/1
  Input1/1 -> Data Type Conversion1/1
  Detect Rise Positive/1 -> Switch/2
  Rem/1 -> Out1/1
  Unit Delay/1 -> Add1/2
  Add1/1 -> Gain2/1, Unit Delay/1

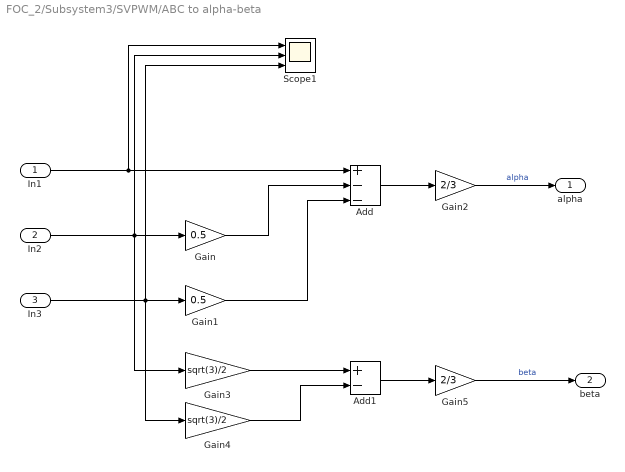
== system FOC_2/Subsystem3/SVPWM/ABC to alpha-beta ==
  In1 : Inport
  In2 : Inport  Port=2
  In3 : Inport  Port=3
  Add : Sum  Inputs=+--
  Add1 : Sum  Inputs=+-
  Gain : Gain  Gain=0.5
  Gain1 : Gain  Gain=0.5
  Gain2 : Gain  Gain=2/3
  Gain3 : Gain  Gain=sqrt(3)/2
  Gain4 : Gain  Gain=sqrt(3)/2
  Gain5 : Gain  Gain=2/3
  Scope1 : Scope  NumInputPorts=3
  alpha : Outport
  beta : Outport  Port=2
  wires:
  Gain3/1 -> Add1/1
  In2/1 -> Gain3/1, Scope1/2, Gain/1
  Gain4/1 -> Add1/2
  Add1/1 -> Gain5/1
  Gain1/1 -> Add/3
  In3/1 -> Scope1/3, Gain4/1, Gain1/1
  Gain/1 -> Add/2
  In1/1 -> Add/1, Scope1/1
  Add/1 -> Gain2/1
  Gain2/1 -> alpha/1  "alpha"
  Gain5/1 -> beta/1  "beta"

== system FOC_2/Subsystem3/SVPWM/PWM ==
  ref1 : Inport
  ref2 : Inport  Port=2
  ref3 : Inport  Port=3
  Carrier : Inport  Port=4
  Relational Operator : RelationalOperator  OutDataTypeStr=boolean  RndMeth=Simplest  InputSameDT=off
  Relational Operator1 : RelationalOperator  OutDataTypeStr=boolean  RndMeth=Simplest  InputSameDT=off
  Relational Operator2 : RelationalOperator  OutDataTypeStr=boolean  RndMeth=Simplest  InputSameDT=off
  PWM1 : Outport
  PWM3 : Outport  Port=2
  PWM5 : Outport  Port=3
  wires:
  ref1/1 -> Relational Operator/1
  ref2/1 -> Relational Operator1/1
  ref3/1 -> Relational Operator2/1
  Carrier/1 -> Relational Operator/2, Relational Operator2/2, Relational Operator1/2
  Relational Operator/1 -> PWM1/1
  Relational Operator1/1 -> PWM3/1
  Relational Operator2/1 -> PWM5/1

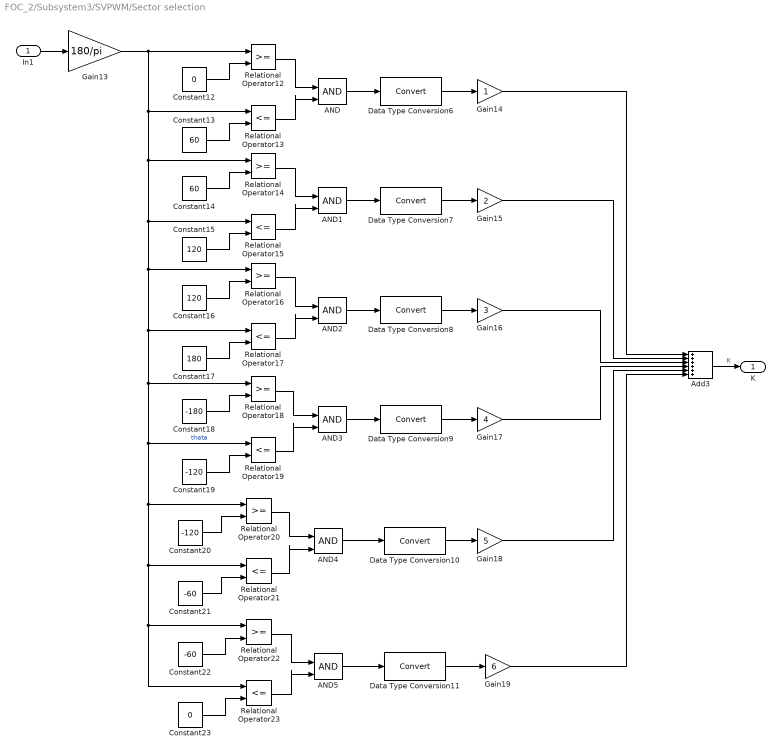
== system FOC_2/Subsystem3/SVPWM/Sector selection ==
  In1 : Inport
  AND{,1..5} (6 alike) : Logic  IconShape=distinctive  AllPortsSameDT=off  OutDataTypeStr=boolean
  Add3 : Sum  Inputs=++++++
  Constant12 : Constant  Value=0
  Constant13 : Constant  Value=60
  Constant14 : Constant  Value=60
  Constant15 : Constant  Value=120
  Constant16 : Constant  Value=120
  Constant17 : Constant  Value=180
  Constant18 : Constant  Value=-180
  Constant19 : Constant  Value=-120
  Constant20 : Constant  Value=-120
  Constant21 : Constant  Value=-60
  Constant22 : Constant  Value=-60
  Constant23 : Constant  Value=0
  Data Type Conversion{6..11} (6 alike) : DataTypeConversion  SaturateOnIntegerOverflow=off  RndMeth=Floor
  Gain13 : Gain  Gain=180/pi
  Gain14 : Gain
  Gain15 : Gain  Gain=2
  Gain16 : Gain  Gain=3
  Gain17 : Gain  Gain=4
  Gain18 : Gain  Gain=5
  Gain19 : Gain  Gain=6
  Relational Operator{12,14,16,18,20,22} (6 alike) : RelationalOperator  OutDataTypeStr=boolean  RndMeth=Simplest  InputSameDT=off
  Relational Operator{13,15,17,19,21,23} (6 alike) : RelationalOperator  Operator=<=  OutDataTypeStr=boolean  RndMeth=Simplest  InputSameDT=off
  K : Outport
  wires:
  AND2/1 -> Data Type Conversion8/1
  Relational Operator14/1 -> AND1/1
  Relational Operator12/1 -> AND/1
  Data Type Conversion10/1 -> Gain18/1
  Data Type Conversion8/1 -> Gain16/1
  Relational Operator19/1 -> AND3/2
  Gain13/1 -> Relational Operator14/1, Relational Operator18/1, Relational Operator19/1, Relational Operator20/1, Relational Operator22/1, Relational Operator23/1, Relational Operator21/1, Relational Operator17/1, Relational Operator16/1, Relational Operator15/1, Relational Operator13/1, Relational Operator12/1  "theta"
  Data Type Conversion6/1 -> Gain14/1
  Constant21/1 -> Relational Operator21/2
  Constant19/1 -> Relational Operator19/2
  Gain19/1 -> Add3/6
  Constant18/1 -> Relational Operator18/2
  AND4/1 -> Data Type Conversion10/1
  Constant22/1 -> Relational Operator22/2
  Relational Operator22/1 -> AND5/1
  Relational Operator18/1 -> AND3/1
  Gain15/1 -> Add3/2
  Relational Operator23/1 -> AND5/2
  Data Type Conversion11/1 -> Gain19/1
  Constant16/1 -> Relational Operator16/2
  Data Type Conversion7/1 -> Gain15/1
  Constant23/1 -> Relational Operator23/2
  Relational Operator20/1 -> AND4/1
  Gain18/1 -> Add3/5
  Gain14/1 -> Add3/1
  AND1/1 -> Data Type Conversion7/1
  Constant14/1 -> Relational Operator14/2
  Relational Operator16/1 -> AND2/1
  Relational Operator17/1 -> AND2/2
  Gain17/1 -> Add3/4
  Constant12/1 -> Relational Operator12/2
  Gain16/1 -> Add3/3
  Relational Operator13/1 -> AND/2
  Relational Operator15/1 -> AND1/2
  Data Type Conversion9/1 -> Gain17/1
  AND/1 -> Data Type Conversion6/1
  Constant13/1 -> Relational Operator13/2
  Relational Operator21/1 -> AND4/2
  AND3/1 -> Data Type Conversion9/1
  Constant20/1 -> Relational Operator20/2
  Constant17/1 -> Relational Operator17/2
  AND5/1 -> Data Type Conversion11/1
  Constant15/1 -> Relational Operator15/2
  Add3/1 -> K/1  "K"
  In1/1 -> Gain13/1

== system FOC_2/Subsystem3/SVPWM/Subsystem3 ==
  In1 : Inport
  In2 : Inport  Port=2
  In3 : Inport  Port=3
  Add10 : Sum
  Add8 : Sum  Inputs=+++
  Add9 : Sum
  Gain{9..12} (4 alike) : Gain  Gain=0.5
  S1 : Outport
  S3 : Outport  Port=2
  S6 : Outport  Port=3
  S5 : Outport  Port=4
  wires:
  In3/1 -> Gain9/1, Gain10/1, Gain12/1, Gain11/1
  Gain11/1 -> Add10/2
  Gain9/1 -> Add8/3
  Gain10/1 -> Add9/2
  Add8/1 -> S1/1  "S1"
  In2/1 -> Add9/1, Add8/2
  In1/1 -> Add10/1, Add8/1
  Add9/1 -> S3/1  "S3"
  Gain12/1 -> S5/1  "S5"
  Add10/1 -> S6/1  "S6"

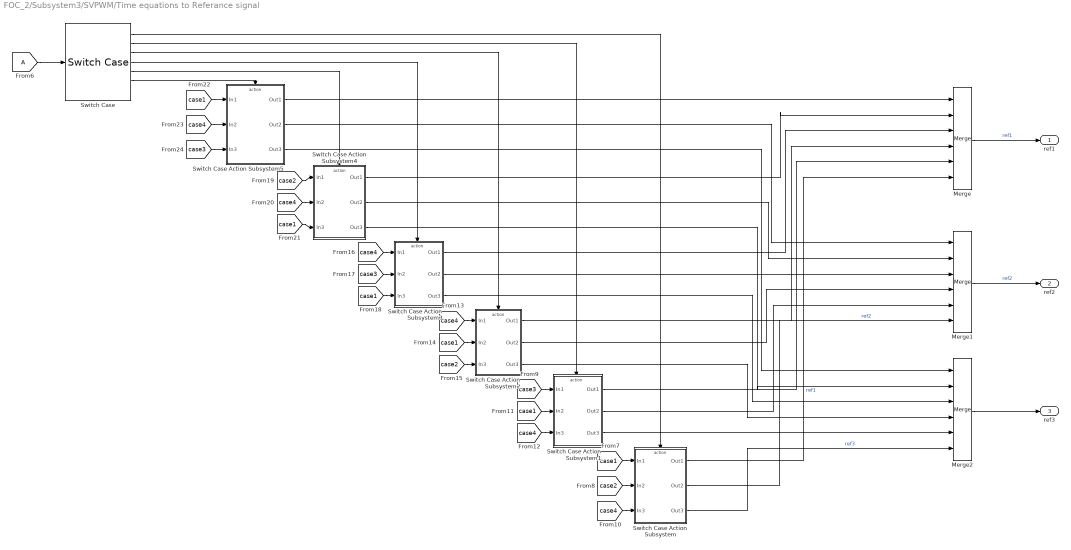
== system FOC_2/Subsystem3/SVPWM/Time equations to Referance signal ==
  From6 : From  TagVisibility=global
  Merge : Merge  Inputs=6
  Merge1 : Merge  Inputs=6
  Merge2 : Merge  Inputs=6
  Switch Case : SwitchCase  CaseConditions={1 2 3 4 5 6}
  Switch Case Action Subsystem : Subsystem  TreatAsAtomicUnit=on
  Switch Case Action Subsystem1 : Subsystem  TreatAsAtomicUnit=on
  Switch Case Action Subsystem2 : Subsystem  TreatAsAtomicUnit=on
  Switch Case Action Subsystem3 : Subsystem  TreatAsAtomicUnit=on
  Switch Case Action Subsystem4 : Subsystem  TreatAsAtomicUnit=on
  Switch Case Action Subsystem5 : Subsystem  TreatAsAtomicUnit=on
  ref1 : Outport
  "ref2 " : Outport  Port=2
  ref3 : Outport  Port=3
  wires:
  [case3] -> Switch Case Action Subsystem5/3(In3)
  Switch Case Action Subsystem4/1(Out1) -> Merge/2
  [case1] -> Switch Case Action Subsystem2/2(In2)
  Switch Case Action Subsystem3/2(Out2) -> Merge1/3
  [case4] -> Switch Case Action Subsystem3/1(In1)
  Switch Case/4 -> Switch Case Action Subsystem3/Action
  [case2] -> Switch Case Action Subsystem4/1(In1)
  Switch Case/6 -> Switch Case Action Subsystem5/Action
  [case4] -> Switch Case Action Subsystem1/3(In3)
  [case1] -> Switch Case Action Subsystem5/1(In1)
  [case3] -> Switch Case Action Subsystem1/1(In1)
  Merge/1 -> ref1/1  "ref1"
  Switch Case Action Subsystem5/1(Out1) -> Merge/1
  Switch Case/5 -> Switch Case Action Subsystem4/Action
  Switch Case Action Subsystem4/3(Out3) -> Merge2/2
  [case1] -> Switch Case Action Subsystem/1(In1)
  Switch Case Action Subsystem2/3(Out3) -> Merge2/4
  Switch Case Action Subsystem4/2(Out2) -> Merge1/2
  Switch Case/3 -> Switch Case Action Subsystem2/Action
  Switch Case Action Subsystem/2(Out2) -> Merge1/6  "ref2"
  Switch Case Action Subsystem3/3(Out3) -> Merge2/3
  Switch Case Action Subsystem5/2(Out2) -> Merge1/1
  [case3] -> Switch Case Action Subsystem3/2(In2)
  Switch Case/2 -> Switch Case Action Subsystem1/Action
  Switch Case Action Subsystem2/1(Out1) -> Merge/4
  Switch Case Action Subsystem2/2(Out2) -> Merge1/4
  [case1] -> Switch Case Action Subsystem4/3(In3)
  [case4] -> Switch Case Action Subsystem5/2(In2)
  Switch Case/1 -> Switch Case Action Subsystem/Action
  Switch Case Action Subsystem5/3(Out3) -> Merge2/1
  [case4] -> Switch Case Action Subsystem2/1(In1)
  Switch Case Action Subsystem3/1(Out1) -> Merge/3
  [case4] -> Switch Case Action Subsystem/3(In3)
  Merge2/1 -> ref3/1
  From6/1 -> Switch Case/1
  [case4] -> Switch Case Action Subsystem4/2(In2)
  [case2] -> Switch Case Action Subsystem/2(In2)
  [case2] -> Switch Case Action Subsystem2/3(In3)
  [case1] -> Switch Case Action Subsystem3/3(In3)
  Switch Case Action Subsystem1/2(Out2) -> Merge1/5
  Switch Case Action Subsystem/1(Out1) -> Merge/6  "ref1"
  Switch Case Action Subsystem1/1(Out1) -> Merge/5
  Switch Case Action Subsystem/3(Out3) -> Merge2/6  "ref3"
  Switch Case Action Subsystem1/3(Out3) -> Merge2/5
  [case1] -> Switch Case Action Subsystem1/2(In2)
  Merge1/1 -> "ref2 "/1  "ref2"

== system FOC_2/Subsystem3/SVPWM/polar form ==
  In1 : Inport
  In2 : Inport  Port=2
  Add2 : Sum
  Atan2 : Trigonometry  Operator=atan2
  Math Function : Math  Operator=square  SignedPower=on
  Math Function1 : Math  Operator=square  SignedPower=on
  Saturation2 : Saturate  UpperLimit=0.95 * Vdc /sqrt(3)  LowerLimit=0
  Scope1 : Scope  NumInputPorts=2
  Scope2 : Scope  NumInputPorts=2
  Square Root : Sqrt
  Vr : Outport
  Angle : Outport  Port=2
  wires:
  In2/1 -> Scope2/2, Atan2/2, Math Function1/1
  In1/1 -> Scope2/1, Atan2/1, Math Function/1
  Math Function1/1 -> Add2/2
  Add2/1 -> Square Root/1
  Math Function/1 -> Add2/1
  Atan2/1 -> Angle/1
  Square Root/1 -> Saturation2/1, Scope1/1  "Vr"
  Saturation2/1 -> Vr/1, Scope1/2

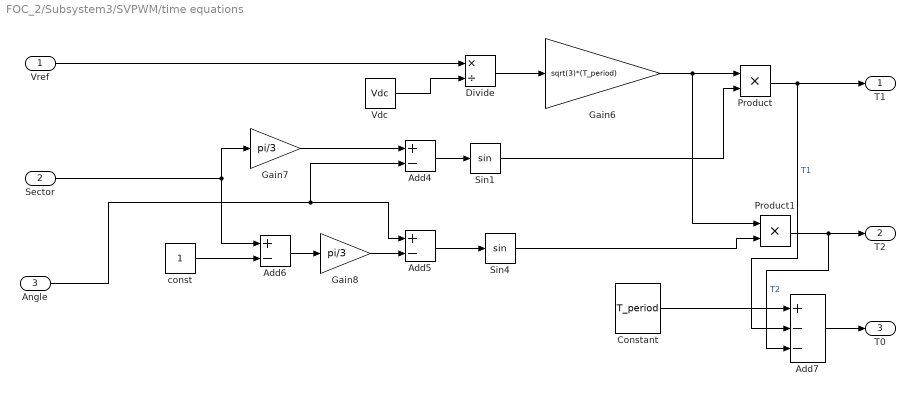
== system FOC_2/Subsystem3/SVPWM/time equations ==
  Vref : Inport
  Sector : Inport  Port=2
  Angle : Inport  Port=3
  Add4 : Sum  Inputs=+-
  Add5 : Sum  Inputs=+-
  Add6 : Sum  Inputs=+-
  Add7 : Sum  Inputs=+--
  Constant : Constant  Value=T_period
  Divide : Product  Inputs=*/
  Gain6 : Gain  Gain=sqrt(3)*(T_period)
  Gain7 : Gain  Gain=pi/3
  Gain8 : Gain  Gain=pi/3
  Product : Product
  Product1 : Product
  Sin1 : Trigonometry
  Sin4 : Trigonometry
  Vdc : Constant  Value=Vdc
  const : Constant
  T1 : Outport
  T2 : Outport  Port=2
  T0 : Outport  Port=3
  wires:
  Vdc/1 -> Divide/2
  Gain6/1 -> Product1/1, Product/1
  Divide/1 -> Gain6/1
  Add6/1 -> Gain8/1
  Constant/1 -> Add7/1
  Gain7/1 -> Add4/1
  Add5/1 -> Sin4/1
  Sin4/1 -> Product1/2
  Sin1/1 -> Product/2
  Gain8/1 -> Add5/2
  Angle/1 -> Add5/1, Add4/2
  const/1 -> Add6/2
  Product1/1 -> T2/1, Add7/3  "T2"
  Sector/1 -> Gain7/1, Add6/1
  Add4/1 -> Sin1/1
  Vref/1 -> Divide/1
  Product/1 -> Add7/2, T1/1  "T1"
  Add7/1 -> T0/1

== system FOC_2/Subsystem3/Subsystem2/PI_Controller_Id ==
  Id_error : Inport
  Discrete-Time Integrator1 : DiscreteIntegrator  SampleTime=-1  ICPrevOutput=DiscIntNeverNeededParam  ICPrevScaledInput=DiscIntNeverNeededParam
  Gain1 : Gain  Gain=Kp
  Gain2 : Gain  Gain=Ki
  Product : Product
  Scope : Scope  NumInputPorts=2
  Scope1 : Scope
  Sum1 : Sum
  Vd_coupled : Outport
  wires:
  [Stop_d_integrator] -> Scope/2, Product/1
  Sum1/1 -> Scope1/1, Vd_coupled/1
  Product/1 -> Scope/1, Discrete-Time Integrator1/1
  Gain2/1 -> Product/2
  Discrete-Time Integrator1/1 -> Sum1/2
  Gain1/1 -> Sum1/1
  Id_error/1 -> Gain2/1, Gain1/1

== system FOC_2/Subsystem3/Subsystem2/PI_Controller_Iq ==
  Iq_error : Inport
  Discrete-Time Integrator1 : DiscreteIntegrator  SampleTime=-1  ICPrevOutput=DiscIntNeverNeededParam  ICPrevScaledInput=DiscIntNeverNeededParam
  Gain1 : Gain  Gain=Kp
  Gain2 : Gain  Gain=Ki
  Product : Product
  Scope : Scope  NumInputPorts=2
  Scope1 : Scope
  Sum1 : Sum
  Vq_coupled : Outport
  wires:
  Product/1 -> Scope/1, Discrete-Time Integrator1/1
  Iq_error/1 -> Gain2/1, Gain1/1
  Discrete-Time Integrator1/1 -> Sum1/2
  Gain1/1 -> Sum1/1
  Gain2/1 -> Product/2
  [Stop_q_integrator] -> Scope/2, Product/1
  Sum1/1 -> Scope1/1, Vq_coupled/1

== system FOC_2/Subsystem3/Subsystem5/Limitations ==
  Vq_ref1 : Inport
  Vd_ref1 : Inport  Port=2
  Action Port : ActionPort  ActionPortLabel=else
  Add : Sum
  Gain : Gain  Gain=sqrt(3)
  Gain1 : Gain  Gain=Vdc*ma
  Gain2 : Gain  Gain=Vdc*ma
  Product : Product  Inputs=*/
  Product1 : Product  Inputs=/*
  Sqrt : Sqrt
  Square : Math  Operator=square  SignedPower=on
  Square1 : Math  Operator=square  SignedPower=on
  Vq_ref2 : Outport
  Vd_ref2 : Outport  Port=2
  wires:
  Vq_ref1/1 -> Gain2/1, Square/1
  Vd_ref1/1 -> Gain1/1, Square1/1
  Square/1 -> Add/1
  Square1/1 -> Add/2
  Add/1 -> Sqrt/1
  Sqrt/1 -> Gain/1
  Gain2/1 -> Product/1
  Gain1/1 -> Product1/2
  Gain/1 -> Product/2, Product1/1
  Product/1 -> Vq_ref2/1
  Product1/1 -> Vd_ref2/1

== system FOC_2/Subsystem3/Subsystem5/Linear Operation  ==
  Vq_ref1 : Inport
  Vd_ref1 : Inport  Port=2
  Action Port : ActionPort  ActionPortLabel=if(u1 <= 0)
  Vq_ref2 : Outport
  Vd_ref2 : Outport  Port=2
  wires:
  Vq_ref1/1 -> Vq_ref2/1
  Vd_ref1/1 -> Vd_ref2/1

== system FOC_2/Subsystem3/SVPWM/Time equations to Referance signal/Switch Case Action Subsystem ==
  In1 : Inport
  In2 : Inport  Port=2
  In3 : Inport  Port=3
  Action Port : ActionPort  ActionPortLabel=case [ 1 ]:
  Out1 : Outport
  Out2 : Outport  Port=2
  Out3 : Outport  Port=3
  wires:
  In1/1 -> Out1/1
  In2/1 -> Out2/1
  In3/1 -> Out3/1

== system FOC_2/Subsystem3/SVPWM/Time equations to Referance signal/Switch Case Action Subsystem1 ==
  In1 : Inport
  In2 : Inport  Port=2
  In3 : Inport  Port=3
  Action Port : ActionPort  ActionPortLabel=case [ 2 ]:
  Out1 : Outport
  Out2 : Outport  Port=2
  Out3 : Outport  Port=3
  wires:
  In1/1 -> Out1/1
  In2/1 -> Out2/1
  In3/1 -> Out3/1

== system FOC_2/Subsystem3/SVPWM/Time equations to Referance signal/Switch Case Action Subsystem2 ==
  In1 : Inport
  In2 : Inport  Port=2
  In3 : Inport  Port=3
  Action Port : ActionPort  ActionPortLabel=case [ 3 ]:
  Out1 : Outport
  Out2 : Outport  Port=2
  Out3 : Outport  Port=3
  wires:
  In1/1 -> Out1/1
  In2/1 -> Out2/1
  In3/1 -> Out3/1

== system FOC_2/Subsystem3/SVPWM/Time equations to Referance signal/Switch Case Action Subsystem3 ==
  In1 : Inport
  In2 : Inport  Port=2
  In3 : Inport  Port=3
  Action Port : ActionPort  ActionPortLabel=case [ 4 ]:
  Out1 : Outport
  Out2 : Outport  Port=2
  Out3 : Outport  Port=3
  wires:
  In1/1 -> Out1/1
  In2/1 -> Out2/1
  In3/1 -> Out3/1

== system FOC_2/Subsystem3/SVPWM/Time equations to Referance signal/Switch Case Action Subsystem4 ==
  In1 : Inport
  In2 : Inport  Port=2
  In3 : Inport  Port=3
  Action Port : ActionPort  ActionPortLabel=case [ 5 ]:
  Out1 : Outport
  Out2 : Outport  Port=2
  Out3 : Outport  Port=3
  wires:
  In1/1 -> Out1/1
  In2/1 -> Out2/1
  In3/1 -> Out3/1

== system FOC_2/Subsystem3/SVPWM/Time equations to Referance signal/Switch Case Action Subsystem5 ==
  In1 : Inport
  In2 : Inport  Port=2
  In3 : Inport  Port=3
  Action Port : ActionPort  ActionPortLabel=case [ 6 ]:
  Out1 : Outport
  Out2 : Outport  Port=2
  Out3 : Outport  Port=3
  wires:
  In1/1 -> Out1/1
  In2/1 -> Out2/1
  In3/1 -> Out3/1
